simulink model "TempMeasure"  (R2014a)
settings: configuration reference "AR_Drone_ConfigSet" (kept outside this file)
libraries: simulink x6, AR_Drone_2_Library x2
settings Model: SimulationMode=external  ExtModeTrigDuration=480000  Creator=darenlee  LastModifiedBy=darenlee

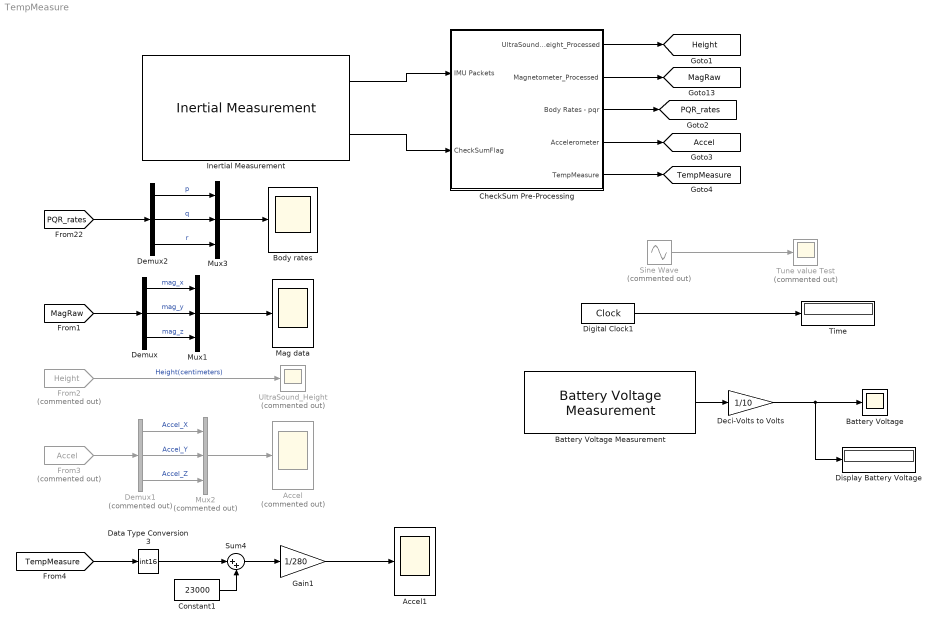
== system TempMeasure ==
  Accel : Scope  Commented=on
      settings: ShowLegends=on  TimeRange=100  YMin=2000  YMax=2550  SaveName=Accel
  Accel1 : Scope
      settings: ShowLegends=on  TimeRange=200  YMin=39  YMax=43.5  SaveName=TempMeasure
  Battery Voltage : Scope
      settings: YMin=12.3575  YMax=12.4  SaveName=Voltage_Measure
  Battery Voltage Measurement : AR_Drone_2_Library/Battery Voltage Measurement  SFunctionSpec=void BatteryMeasure_step(single y1[1])  SampleTime=0.01
  Body rates : Scope
      settings: ShowLegends=on  TimeRange=200  YMin=-45  YMax=45  SaveName=Gyro
  CheckSum Pre-Processing : Subsystem
  Constant1 : Constant  Value=23000  OutDataTypeStr=int16
  Data Type Conversion3 : DataTypeConversion  OutDataTypeStr=int16
  Deci-Volts to Volts : Gain  Gain=1/10
  Demux : Demux  Outputs=3
  Demux1 : Demux  Commented=on  Outputs=3
  Demux2 : Demux  Outputs=3
  Digital Clock1 : DigitalClock  SampleTime=0.1
  Display Battery Voltage : Display
  From2 : From  Commented=on  GotoTag=Height  TagVisibility=global
  From3 : From  Commented=on  GotoTag=Accel  TagVisibility=global
  Gain1 : Gain  Gain=1/280  OutDataTypeStr=double
  Inertial Measurement : AR_Drone_2_Library/Inertial Measurement  Ts=1/400
  Mag data : Scope
      settings: ShowLegends=on  TimeRange=100  YMin=-125  YMax=150  SaveName=MagData
  Mux1 : Mux  Inputs=3
  Mux2 : Mux  Commented=on  Inputs=3
  Mux3 : Mux  Inputs=3
  Sine Wave : Sin  Commented=on  SineType=Sample based  Amplitude=6  Bias=-1  Samples=1000  SampleTime=0.01
  Sum4 : Sum  Inputs=|++
  Time : Display
  Tune value Test : Scope  Commented=on
      settings: YMin=-35  SaveName=UltraSound_Measure2
  UltraSound_Height : Scope  Commented=on
      settings: YMin=0  YMax=18
  tag scope: Accel=global, Height=global, MagRaw=global, PQR_rates=global, TempMeasure=global
  wires:
  Sine Wave/1 -> Tune value Test/1
  Digital Clock1/1 -> Time/1
  Inertial Measurement/1 -> CheckSum Pre-Processing/1(IMU Packets)
  Inertial Measurement/2 -> CheckSum Pre-Processing/2(CheckSumFlag)
  [MagRaw] -> Demux/1
  Demux/1 -> Mux1/1  "mag_x"
  Demux/2 -> Mux1/2  "mag_y"
  Demux/3 -> Mux1/3  "mag_z"
  Mux1/1 -> Mag data/1
  CheckSum Pre-Processing/1(UltraSoundHeight_Processed) -> [Height]
  Demux2/1 -> Mux3/1  "p"
  Demux2/2 -> Mux3/2  "q"
  Mux3/1 -> Body rates/1
  Demux2/3 -> Mux3/3  "r"
  [PQR_rates] -> Demux2/1
  From2/1 -> UltraSound_Height/1  "Height(centimeters)"
  Demux1/1 -> Mux2/1  "Accel_X"
  Demux1/2 -> Mux2/2  "Accel_Y"
  Mux2/1 -> Accel/1
  Demux1/3 -> Mux2/3  "Accel_Z"
  From3/1 -> Demux1/1
  CheckSum Pre-Processing/4(Accelerometer) -> [Accel]
  CheckSum Pre-Processing/3(Body Rates - pqr) -> [PQR_rates]
  CheckSum Pre-Processing/2(Magnetometer_Processed) -> [MagRaw]
  Battery Voltage Measurement/1 -> Deci-Volts to Volts/1
  Deci-Volts to Volts/1 -> Display Battery Voltage/1, Battery Voltage/1
  CheckSum Pre-Processing/5(TempMeasure) -> [TempMeasure]
  Data Type Conversion3/1 -> Sum4/1
  Constant1/1 -> Sum4/2
  Sum4/1 -> Gain1/1
  Gain1/1 -> Accel1/1
  [TempMeasure] -> Data Type Conversion3/1

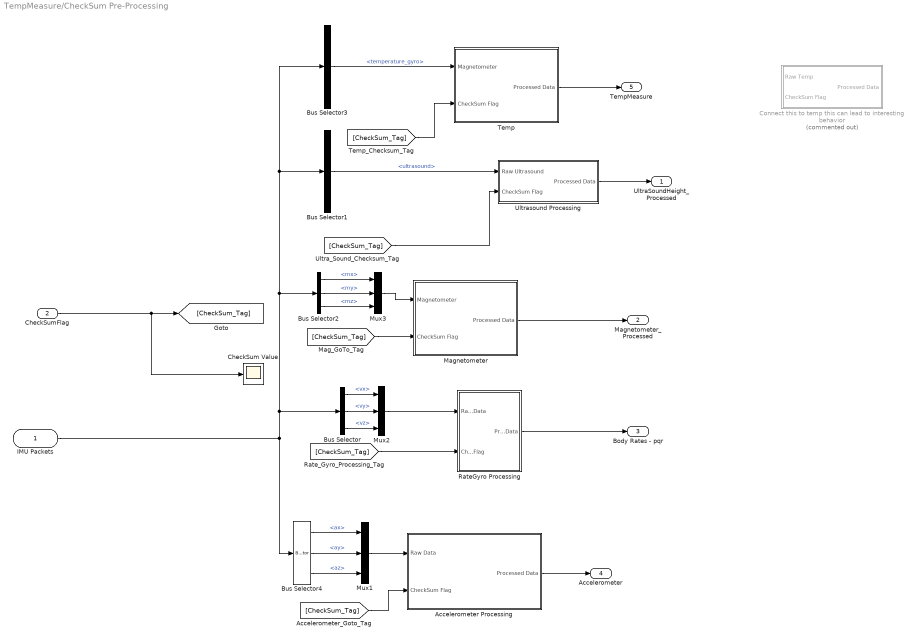
== system TempMeasure/CheckSum Pre-Processing ==
  IMU Packets : Inport
  CheckSumFlag : Inport  Port=2
  Accelerometer Processing : Subsystem
  Bus Selector : BusSelector  OutputSignals=vx,vy,vz
  Bus Selector1 : BusSelector  OutputSignals=ultrasound
  Bus Selector2 : BusSelector  OutputSignals=mx,my,mz
  Bus Selector3 : BusSelector  OutputSignals=temperature_gyro
  Bus Selector4 : BusSelector  OutputSignals=ax,ay,az
  CheckSum Value : Scope
      settings: YMin=0  YMax=2500  SaveName=CheckSum
  Connect this to temp this can lead to interesting behavior : Subsystem  Commented=on
  Magnetometer : Subsystem
  Mux1 : Mux  Inputs=3
  Mux2 : Mux  Inputs=3
  Mux3 : Mux  Inputs=3
  RateGyro Processing : Subsystem
  Temp : Subsystem
  Ultrasound Processing : Subsystem
  UltraSoundHeight_Processed : Outport
  Magnetometer_Processed : Outport  Port=2
  Body Rates - pqr : Outport  Port=3
  Accelerometer : Outport  Port=4
  TempMeasure : Outport  Port=5
  wires:
  Bus Selector1/1 -> Ultrasound Processing/1(Raw Ultrasound)  "<ultrasound>"
  CheckSumFlag/1 -> [CheckSum_Tag], CheckSum Value/1
  IMU Packets/1 -> Bus Selector/1, Bus Selector3/1, Bus Selector1/1, Bus Selector2/1, Bus Selector4/1
  Bus Selector4/1 -> Mux1/1  "<ax>"
  Bus Selector4/2 -> Mux1/2  "<ay>"
  Bus Selector4/3 -> Mux1/3  "<az>"
  Mux1/1 -> Accelerometer Processing/1(Raw Data)
  [CheckSum_Tag] -> Ultrasound Processing/2(CheckSum Flag)
  Accelerometer Processing/1(Processed Data) -> Accelerometer/1
  Bus Selector/1 -> Mux2/1  "<vx>"
  Bus Selector/2 -> Mux2/2  "<vy>"
  Bus Selector/3 -> Mux2/3  "<vz>"
  Mux2/1 -> RateGyro Processing/1(Raw Data)
  [CheckSum_Tag] -> RateGyro Processing/2(CheckSum Flag)
  RateGyro Processing/1(Processed Data) -> Body Rates - pqr/1
  Bus Selector2/1 -> Mux3/1  "<mx>"
  Bus Selector2/2 -> Mux3/2  "<my>"
  Bus Selector2/3 -> Mux3/3  "<mz>"
  Mux3/1 -> Magnetometer/1(Magnetometer)
  [CheckSum_Tag] -> Magnetometer/2(CheckSum Flag)
  Magnetometer/1(Processed Data) -> Magnetometer_Processed/1
  [CheckSum_Tag] -> Accelerometer Processing/2(CheckSum Flag)
  Ultrasound Processing/1(Processed Data) -> UltraSoundHeight_Processed/1
  Bus Selector3/1 -> Temp/1(Magnetometer)  "<temperature_gyro>"
  ? -> Connect this to temp this can lead to interesting behavior/2(CheckSum Flag)
  [CheckSum_Tag] -> Temp/2(CheckSum Flag)
  Temp/1(Processed Data) -> TempMeasure/1

== system TempMeasure/CheckSum Pre-Processing/Accelerometer Processing ==
  Raw Data : Inport
  CheckSum Flag : Inport  Port=2
  Calculate Accel Data : Subsystem  Commented=through
  CheckSum Correction : Subsystem
  Processed Data : Outport
  wires:
  CheckSum Flag/1 -> CheckSum Correction/2(CheckSumFlag)
  Raw Data/1 -> Calculate Accel Data/1(Raw Accel Data)
  CheckSum Correction/1(Pre-Processed Height) -> Processed Data/1
  Calculate Accel Data/1(Processed Accel Data) -> CheckSum Correction/1(CalculatedData)

== system TempMeasure/CheckSum Pre-Processing/Connect this to temp this can lead to interesting behavior ==
  note: '192.168.1.1' 1 17725
  Raw Temp : Inport
  CheckSum Flag : Inport  Port=2
  CheckSum Correction : Subsystem
  Display : Display
  Saturation1 : Saturate  UpperLimit=100e3  LowerLimit=0
  Processed Data : Outport
  wires:
  Raw Temp/1 -> CheckSum Correction/1(CalculatedData)
  CheckSum Flag/1 -> CheckSum Correction/2(CheckSumFlag)
  CheckSum Correction/1(Pre-Processed Height) -> Display/1, Saturation1/1
  Saturation1/1 -> Processed Data/1

== system TempMeasure/CheckSum Pre-Processing/Magnetometer ==
  Magnetometer : Inport
  CheckSum Flag : Inport  Port=2
  CheckSum Correction : Subsystem
  Display : Display
  Process Raw Mag Data : Subsystem  Commented=through
  Processed Data : Outport
  wires:
  CheckSum Flag/1 -> CheckSum Correction/2(CheckSumFlag)
  CheckSum Correction/1(Pre-Processed Data) -> Display/1, Processed Data/1
  Magnetometer/1 -> Process Raw Mag Data/1(Magnetometer)
  Process Raw Mag Data/1(ProcessedData) -> CheckSum Correction/1(CalculatedData)

== system TempMeasure/CheckSum Pre-Processing/RateGyro Processing ==
  Raw Data : Inport
  CheckSum Flag : Inport  Port=2
  CheckSum Correction : Subsystem
  Process Data : Subsystem  Commented=through
  Processed Data : Outport
  wires:
  CheckSum Flag/1 -> CheckSum Correction/2(CheckSumFlag)
  CheckSum Correction/1(Pre-Processed Height) -> Processed Data/1
  Raw Data/1 -> Process Data/1(Raw Data)
  Process Data/1(Processed Data) -> CheckSum Correction/1(CalculatedData)

== system TempMeasure/CheckSum Pre-Processing/Temp ==
  Magnetometer : Inport
  CheckSum Flag : Inport  Port=2
  CheckSum Correction : Subsystem
  Display : Display
  Process Raw Mag Data : Subsystem  Commented=through
  Processed Data : Outport
  wires:
  CheckSum Flag/1 -> CheckSum Correction/2(CheckSumFlag)
  CheckSum Correction/1(Pre-Processed Data) -> Display/1, Processed Data/1
  Magnetometer/1 -> Process Raw Mag Data/1(Magnetometer)
  Process Raw Mag Data/1(ProcessedData) -> CheckSum Correction/1(CalculatedData)

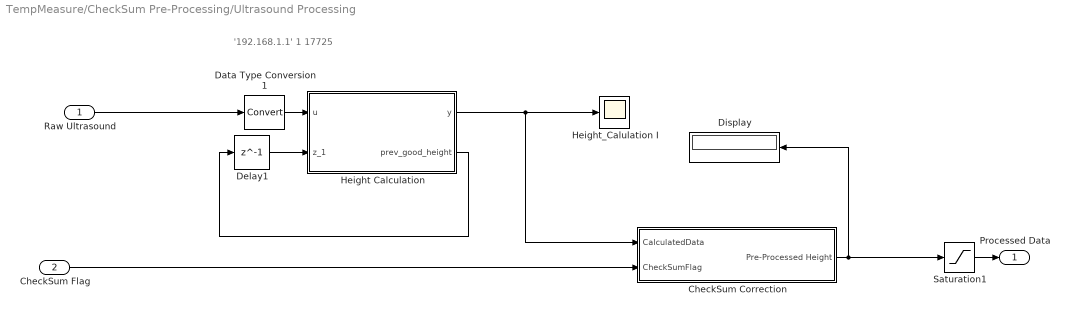
== system TempMeasure/CheckSum Pre-Processing/Ultrasound Processing ==
  note: '192.168.1.1' 1 17725
  Raw Ultrasound : Inport
  CheckSum Flag : Inport  Port=2
  CheckSum Correction : Subsystem
  Data Type Conversion1 : DataTypeConversion
  Delay1 : Delay  DelayLength=1  InitialCondition=0
  Display : Display
  Height Calculation : MATLAB Function  TreatAsAtomicUnit=on
  Height_Calulation I : Scope
      settings: TimeRange=622.5296442687759  YMin=0  YMax=300  SaveName=CalculatedHeight
  Saturation1 : Saturate  UpperLimit=100e3  LowerLimit=0
  Processed Data : Outport
  wires:
  Delay1/1 -> Height Calculation/2(z_1)
  Data Type Conversion1/1 -> Height Calculation/1(u)
  Height Calculation/2(prev_good_height) -> Delay1/1
  Raw Ultrasound/1 -> Data Type Conversion1/1
  Height Calculation/1(y) -> CheckSum Correction/1(CalculatedData), Height_Calulation I/1
  CheckSum Flag/1 -> CheckSum Correction/2(CheckSumFlag)
  CheckSum Correction/1(Pre-Processed Height) -> Display/1, Saturation1/1
  Saturation1/1 -> Processed Data/1

== system TempMeasure/CheckSum Pre-Processing/Accelerometer Processing/Calculate Accel Data ==
  Raw Accel Data : Inport
  Bias : Constant  Value=[0 4096 4096]
  Gain : Gain  Gain=[0.001953125, 0.001953125, 0.001953125]
  Neutral Bias : Constant  Value=[2048 2048 2048]
  Sum : Sum  Inputs=|-+
  Sum1 : Sum  Inputs=|+-
  Processed Accel Data : Outport
  wires:
  Raw Accel Data/1 -> Sum/1
  Sum1/1 -> Gain/1
  Gain/1 -> Processed Accel Data/1
  Sum/1 -> Sum1/1
  Neutral Bias/1 -> Sum1/2
  Bias/1 -> Sum/2

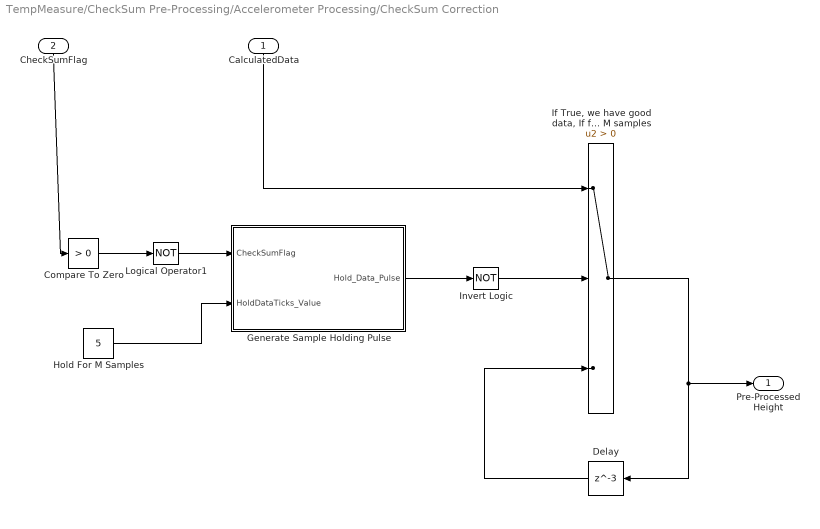
== system TempMeasure/CheckSum Pre-Processing/Accelerometer Processing/CheckSum Correction ==
  CalculatedData : Inport
  CheckSumFlag : Inport  Port=2
  Compare To Zero : simulink/Logic and Bit Operations/Compare To Zero  relop=>  OutDataTypeStr=boolean
  Delay : Delay  DelayLength=3  InitialCondition=0
  Generate Sample Holding Pulse : Subsystem
  Hold For M Samples : Constant  Value=5
  "If True, we have good data, If false, we have bad data, With bad data, use previous good data from N samples ago and hold it on that value for M samples" : Switch  Criteria=u2 > Threshold
  Invert Logic : Logic  Operator=NOT  AllPortsSameDT=off  OutDataTypeStr=boolean
  Logical Operator1 : Logic  Operator=NOT  AllPortsSameDT=off  OutDataTypeStr=boolean
  Pre-Processed Height : Outport
  wires:
  CheckSumFlag/1 -> Compare To Zero/1
  CalculatedData/1 -> "If True, we have good data, If false, we have bad data, With bad data, use previous good data from N samples ago and hold it on that value for M samples"/1
  "If True, we have good data, If false, we have bad data, With bad data, use previous good data from N samples ago and hold it on that value for M samples"/1 -> Pre-Processed Height/1, Delay/1
  Delay/1 -> "If True, we have good data, If false, we have bad data, With bad data, use previous good data from N samples ago and hold it on that value for M samples"/3
  Compare To Zero/1 -> Logical Operator1/1
  Generate Sample Holding Pulse/1(Hold_Data_Pulse) -> Invert Logic/1
  Logical Operator1/1 -> Generate Sample Holding Pulse/1(CheckSumFlag)
  Invert Logic/1 -> "If True, we have good data, If false, we have bad data, With bad data, use previous good data from N samples ago and hold it on that value for M samples"/2
  Hold For M Samples/1 -> Generate Sample Holding Pulse/2(HoldDataTicks_Value)

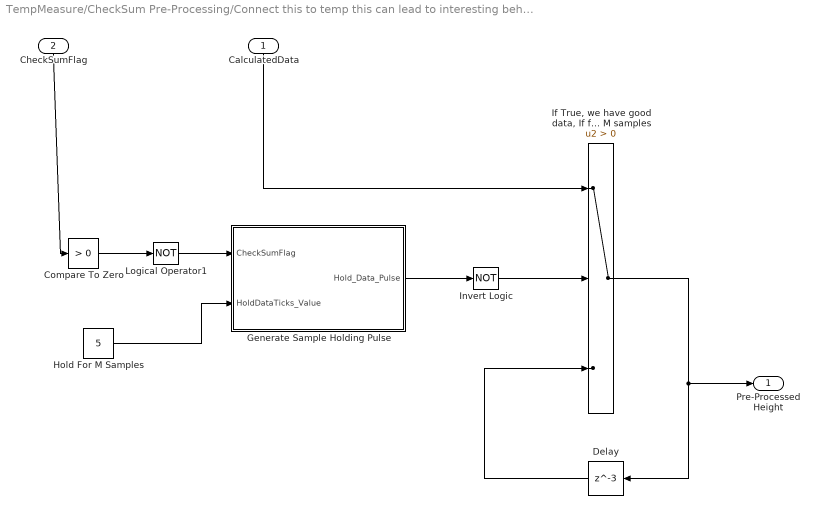
== system TempMeasure/CheckSum Pre-Processing/Connect this to temp this can lead to interesting behavior/CheckSum Correction ==
  CalculatedData : Inport
  CheckSumFlag : Inport  Port=2
  Compare To Zero : simulink/Logic and Bit Operations/Compare To Zero  relop=>  OutDataTypeStr=boolean
  Delay : Delay  DelayLength=3  InitialCondition=0
  Generate Sample Holding Pulse : Subsystem
  Hold For M Samples : Constant  Value=5
  "If True, we have good data, If false, we have bad data, With bad data, use previous good data from N samples ago and hold it on that value for M samples" : Switch  Criteria=u2 > Threshold
  Invert Logic : Logic  Operator=NOT  AllPortsSameDT=off  OutDataTypeStr=boolean
  Logical Operator1 : Logic  Operator=NOT  AllPortsSameDT=off  OutDataTypeStr=boolean
  Pre-Processed Height : Outport
  wires:
  CheckSumFlag/1 -> Compare To Zero/1
  CalculatedData/1 -> "If True, we have good data, If false, we have bad data, With bad data, use previous good data from N samples ago and hold it on that value for M samples"/1
  "If True, we have good data, If false, we have bad data, With bad data, use previous good data from N samples ago and hold it on that value for M samples"/1 -> Pre-Processed Height/1, Delay/1
  Delay/1 -> "If True, we have good data, If false, we have bad data, With bad data, use previous good data from N samples ago and hold it on that value for M samples"/3
  Compare To Zero/1 -> Logical Operator1/1
  Generate Sample Holding Pulse/1(Hold_Data_Pulse) -> Invert Logic/1
  Logical Operator1/1 -> Generate Sample Holding Pulse/1(CheckSumFlag)
  Invert Logic/1 -> "If True, we have good data, If false, we have bad data, With bad data, use previous good data from N samples ago and hold it on that value for M samples"/2
  Hold For M Samples/1 -> Generate Sample Holding Pulse/2(HoldDataTicks_Value)

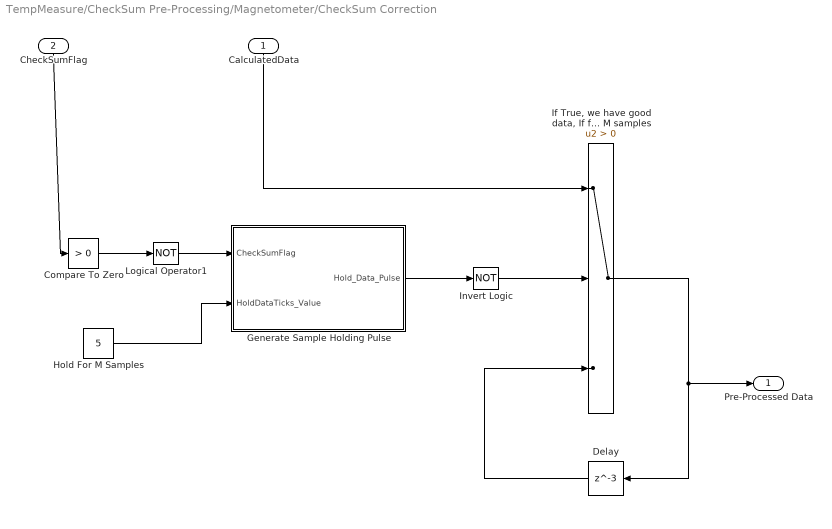
== system TempMeasure/CheckSum Pre-Processing/Magnetometer/CheckSum Correction ==
  CalculatedData : Inport
  CheckSumFlag : Inport  Port=2
  Compare To Zero : simulink/Logic and Bit Operations/Compare To Zero  relop=>  OutDataTypeStr=boolean
  Delay : Delay  DelayLength=3  InitialCondition=0
  Generate Sample Holding Pulse : Subsystem
  Hold For M Samples : Constant  Value=5
  "If True, we have good data, If false, we have bad data, With bad data, use previous good data from N samples ago and hold it on that value for M samples" : Switch  Criteria=u2 > Threshold
  Invert Logic : Logic  Operator=NOT  AllPortsSameDT=off  OutDataTypeStr=boolean
  Logical Operator1 : Logic  Operator=NOT  AllPortsSameDT=off  OutDataTypeStr=boolean
  Pre-Processed Data : Outport
  wires:
  CheckSumFlag/1 -> Compare To Zero/1
  CalculatedData/1 -> "If True, we have good data, If false, we have bad data, With bad data, use previous good data from N samples ago and hold it on that value for M samples"/1
  "If True, we have good data, If false, we have bad data, With bad data, use previous good data from N samples ago and hold it on that value for M samples"/1 -> Pre-Processed Data/1, Delay/1
  Delay/1 -> "If True, we have good data, If false, we have bad data, With bad data, use previous good data from N samples ago and hold it on that value for M samples"/3
  Compare To Zero/1 -> Logical Operator1/1
  Generate Sample Holding Pulse/1(Hold_Data_Pulse) -> Invert Logic/1
  Logical Operator1/1 -> Generate Sample Holding Pulse/1(CheckSumFlag)
  Invert Logic/1 -> "If True, we have good data, If false, we have bad data, With bad data, use previous good data from N samples ago and hold it on that value for M samples"/2
  Hold For M Samples/1 -> Generate Sample Holding Pulse/2(HoldDataTicks_Value)

== system TempMeasure/CheckSum Pre-Processing/Magnetometer/Process Raw Mag Data ==
  note: magnetometer[ 0 ] = - ( float ) navdata.mx ;
      | magnetometer[ 1 ] = ( float ) navdata.my ;
      | magnetometer[ 2 ] = - ( float ) navdata.mz ;
      | const float Sensitivity[ 3 ] = { 0.0071492608 , 0.0070882491 , 0.0074057781 } ;
      | const float Neutral[ 3 ] = { 118.0 , - 65.0 , 110.0 } ;
  Magnetometer : Inport
  Bias : Constant  Value=[ 118.0, -65.0, 110.0 ]
  Sum : Sum  Inputs=|+-
  postGain : Gain  Gain=[0.0071492608, 0.0070882491, 0.0074057781]
  preGain : Gain  Gain=[-1 1 -1]
  ProcessedData : Outport
  wires:
  postGain/1 -> ProcessedData/1
  Magnetometer/1 -> preGain/1
  Sum/1 -> postGain/1
  preGain/1 -> Sum/1
  Bias/1 -> Sum/2

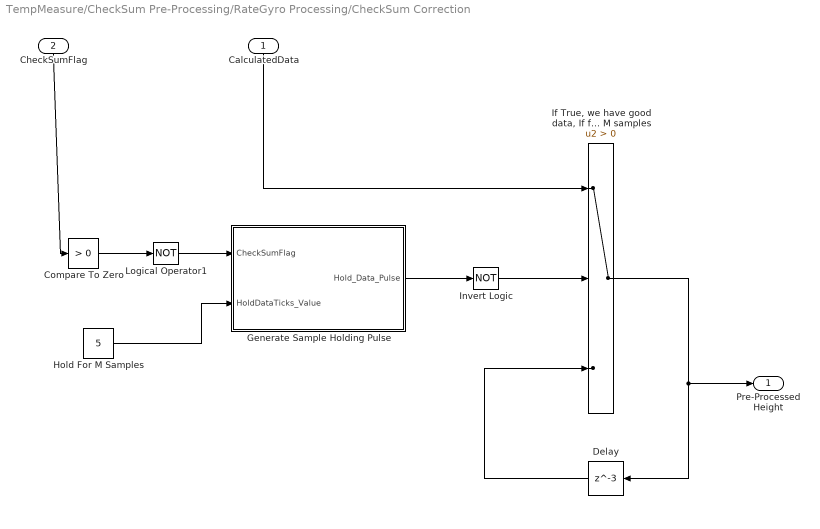
== system TempMeasure/CheckSum Pre-Processing/RateGyro Processing/CheckSum Correction ==
  CalculatedData : Inport
  CheckSumFlag : Inport  Port=2
  Compare To Zero : simulink/Logic and Bit Operations/Compare To Zero  relop=>  OutDataTypeStr=boolean
  Delay : Delay  DelayLength=3  InitialCondition=0
  Generate Sample Holding Pulse : Subsystem
  Hold For M Samples : Constant  Value=5  SampleTime=-1
  "If True, we have good data, If false, we have bad data, With bad data, use previous good data from N samples ago and hold it on that value for M samples" : Switch  Criteria=u2 > Threshold
  Invert Logic : Logic  Operator=NOT  AllPortsSameDT=off  OutDataTypeStr=boolean
  Logical Operator1 : Logic  Operator=NOT  AllPortsSameDT=off  OutDataTypeStr=boolean
  Pre-Processed Height : Outport
  wires:
  CheckSumFlag/1 -> Compare To Zero/1
  CalculatedData/1 -> "If True, we have good data, If false, we have bad data, With bad data, use previous good data from N samples ago and hold it on that value for M samples"/1
  "If True, we have good data, If false, we have bad data, With bad data, use previous good data from N samples ago and hold it on that value for M samples"/1 -> Pre-Processed Height/1, Delay/1
  Delay/1 -> "If True, we have good data, If false, we have bad data, With bad data, use previous good data from N samples ago and hold it on that value for M samples"/3
  Compare To Zero/1 -> Logical Operator1/1
  Generate Sample Holding Pulse/1(Hold_Data_Pulse) -> Invert Logic/1
  Logical Operator1/1 -> Generate Sample Holding Pulse/1(CheckSumFlag)
  Invert Logic/1 -> "If True, we have good data, If false, we have bad data, With bad data, use previous good data from N samples ago and hold it on that value for M samples"/2
  Hold For M Samples/1 -> Generate Sample Holding Pulse/2(HoldDataTicks_Value)

== system TempMeasure/CheckSum Pre-Processing/RateGyro Processing/Process Data ==
  note: const float Sensitivity[ 3 ] = { 0.0609 , 0.0609 , 0.0609 } ;
      | const float Neutral[ 3 ] = { 0.0 , 0.0 , 0.0 } ;
      | const int16_t Offset[ 3 ] = { - 73 , 14 , - 13 } ;
      | const int16_t Noises[ 3 ] = { 35 , 35 , 15 } ;
      |
      | int16_t vRaws[ 3 ] = {
      | Navdata :: IMU :: Gyroscope :: getRawX (),
      | Navdata :: IMU :: Gyroscope :: getRawY (),
      | Navdata :: IMU :: Gyroscope :: getRawZ ()
      | } ;
      |
      | gyroscope[i] = vRaws[i] * Gyroscope :: Sensitivity[i] * M_PI / 180.0 ;
  Raw Data : Inport
  Constant : Constant  Value=[0.0, 0.0, 0.0]
  Gain : Gain  Gain=[0.0609, 0.0609, 0.0609]
  Sum : Sum  Inputs=|++
  Processed Data : Outport
  wires:
  Sum/1 -> Gain/1
  Gain/1 -> Processed Data/1
  Constant/1 -> Sum/2
  Raw Data/1 -> Sum/1

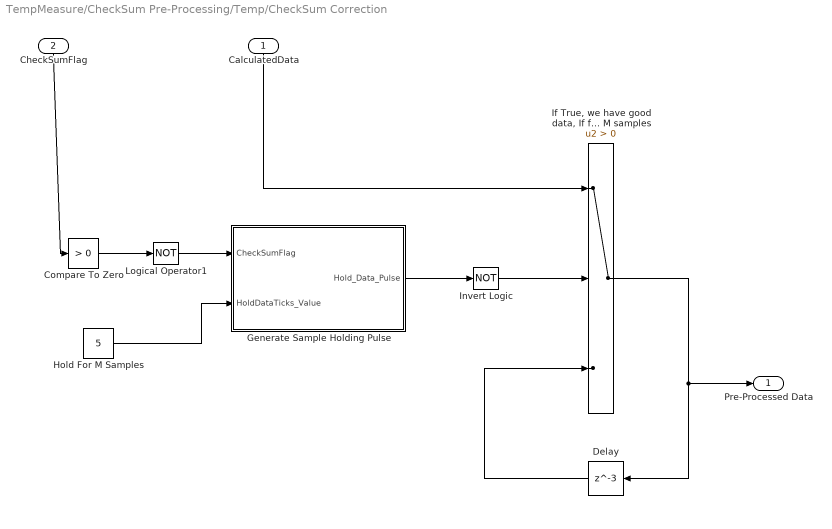
== system TempMeasure/CheckSum Pre-Processing/Temp/CheckSum Correction ==
  CalculatedData : Inport
  CheckSumFlag : Inport  Port=2
  Compare To Zero : simulink/Logic and Bit Operations/Compare To Zero  relop=>  OutDataTypeStr=boolean
  Delay : Delay  DelayLength=3  InitialCondition=0
  Generate Sample Holding Pulse : Subsystem
  Hold For M Samples : Constant  Value=5
  "If True, we have good data, If false, we have bad data, With bad data, use previous good data from N samples ago and hold it on that value for M samples" : Switch  Criteria=u2 > Threshold
  Invert Logic : Logic  Operator=NOT  AllPortsSameDT=off  OutDataTypeStr=boolean
  Logical Operator1 : Logic  Operator=NOT  AllPortsSameDT=off  OutDataTypeStr=boolean
  Pre-Processed Data : Outport
  wires:
  CheckSumFlag/1 -> Compare To Zero/1
  CalculatedData/1 -> "If True, we have good data, If false, we have bad data, With bad data, use previous good data from N samples ago and hold it on that value for M samples"/1
  "If True, we have good data, If false, we have bad data, With bad data, use previous good data from N samples ago and hold it on that value for M samples"/1 -> Pre-Processed Data/1, Delay/1
  Delay/1 -> "If True, we have good data, If false, we have bad data, With bad data, use previous good data from N samples ago and hold it on that value for M samples"/3
  Compare To Zero/1 -> Logical Operator1/1
  Generate Sample Holding Pulse/1(Hold_Data_Pulse) -> Invert Logic/1
  Logical Operator1/1 -> Generate Sample Holding Pulse/1(CheckSumFlag)
  Invert Logic/1 -> "If True, we have good data, If false, we have bad data, With bad data, use previous good data from N samples ago and hold it on that value for M samples"/2
  Hold For M Samples/1 -> Generate Sample Holding Pulse/2(HoldDataTicks_Value)

== system TempMeasure/CheckSum Pre-Processing/Temp/Process Raw Mag Data ==
  note: magnetometer[ 0 ] = - ( float ) navdata.mx ;
      | magnetometer[ 1 ] = ( float ) navdata.my ;
      | magnetometer[ 2 ] = - ( float ) navdata.mz ;
      | const float Sensitivity[ 3 ] = { 0.0071492608 , 0.0070882491 , 0.0074057781 } ;
      | const float Neutral[ 3 ] = { 118.0 , - 65.0 , 110.0 } ;
  Magnetometer : Inport
  Bias : Constant  Value=[ 118.0, -65.0, 110.0 ]
  Sum : Sum  Inputs=|+-
  postGain : Gain  Gain=[0.0071492608, 0.0070882491, 0.0074057781]
  preGain : Gain  Gain=[-1 1 -1]
  ProcessedData : Outport
  wires:
  postGain/1 -> ProcessedData/1
  Magnetometer/1 -> preGain/1
  Sum/1 -> postGain/1
  preGain/1 -> Sum/1
  Bias/1 -> Sum/2

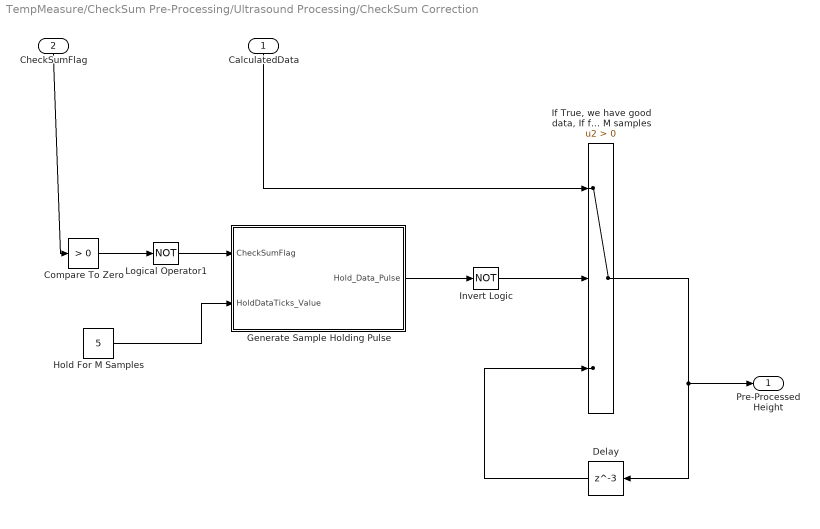
== system TempMeasure/CheckSum Pre-Processing/Ultrasound Processing/CheckSum Correction ==
  CalculatedData : Inport
  CheckSumFlag : Inport  Port=2
  Compare To Zero : simulink/Logic and Bit Operations/Compare To Zero  relop=>  OutDataTypeStr=boolean
  Delay : Delay  DelayLength=3  InitialCondition=0
  Generate Sample Holding Pulse : Subsystem
  Hold For M Samples : Constant  Value=5
  "If True, we have good data, If false, we have bad data, With bad data, use previous good data from N samples ago and hold it on that value for M samples" : Switch  Criteria=u2 > Threshold
  Invert Logic : Logic  Operator=NOT  AllPortsSameDT=off  OutDataTypeStr=boolean
  Logical Operator1 : Logic  Operator=NOT  AllPortsSameDT=off  OutDataTypeStr=boolean
  Pre-Processed Height : Outport
  wires:
  CheckSumFlag/1 -> Compare To Zero/1
  CalculatedData/1 -> "If True, we have good data, If false, we have bad data, With bad data, use previous good data from N samples ago and hold it on that value for M samples"/1
  "If True, we have good data, If false, we have bad data, With bad data, use previous good data from N samples ago and hold it on that value for M samples"/1 -> Pre-Processed Height/1, Delay/1
  Delay/1 -> "If True, we have good data, If false, we have bad data, With bad data, use previous good data from N samples ago and hold it on that value for M samples"/3
  Compare To Zero/1 -> Logical Operator1/1
  Generate Sample Holding Pulse/1(Hold_Data_Pulse) -> Invert Logic/1
  Logical Operator1/1 -> Generate Sample Holding Pulse/1(CheckSumFlag)
  Invert Logic/1 -> "If True, we have good data, If false, we have bad data, With bad data, use previous good data from N samples ago and hold it on that value for M samples"/2
  Hold For M Samples/1 -> Generate Sample Holding Pulse/2(HoldDataTicks_Value)

== system TempMeasure/CheckSum Pre-Processing/Accelerometer Processing/CheckSum Correction/Generate Sample Holding Pulse ==
  CheckSumFlag : Inport
  HoldDataTicks_Value : Inport  Port=2
  Chart : Stateflow chart  TreatAsAtomicUnit=on
  Constant2 : Constant
  Logical Operator1 : Logic  AllPortsSameDT=off  OutDataTypeStr=boolean
  Transition Logic Detection : Subsystem
  Hold_Data_Pulse : Outport
  wires:
  Constant2/1 -> Logical Operator1/1
  Logical Operator1/1 -> Hold_Data_Pulse/1
  Chart/1(output) -> Logical Operator1/2
  Transition Logic Detection/1(Transition Detect) -> Chart/1(if_transition)
  CheckSumFlag/1 -> Transition Logic Detection/1(Input)
  HoldDataTicks_Value/1 -> Chart/2(HoldDataTicks)

== system TempMeasure/CheckSum Pre-Processing/Connect this to temp this can lead to interesting behavior/CheckSum Correction/Generate Sample Holding Pulse ==
  CheckSumFlag : Inport
  HoldDataTicks_Value : Inport  Port=2
  Chart : Stateflow chart  TreatAsAtomicUnit=on
  Constant2 : Constant
  Logical Operator1 : Logic  AllPortsSameDT=off  OutDataTypeStr=boolean
  Transition Logic Detection : Subsystem
  Hold_Data_Pulse : Outport
  wires:
  Constant2/1 -> Logical Operator1/1
  Logical Operator1/1 -> Hold_Data_Pulse/1
  Chart/1(output) -> Logical Operator1/2
  Transition Logic Detection/1(Transition Detect) -> Chart/1(if_transition)
  CheckSumFlag/1 -> Transition Logic Detection/1(Input)
  HoldDataTicks_Value/1 -> Chart/2(HoldDataTicks)

== system TempMeasure/CheckSum Pre-Processing/Magnetometer/CheckSum Correction/Generate Sample Holding Pulse ==
  CheckSumFlag : Inport
  HoldDataTicks_Value : Inport  Port=2
  Chart : Stateflow chart  TreatAsAtomicUnit=on
  Constant2 : Constant
  Logical Operator1 : Logic  AllPortsSameDT=off  OutDataTypeStr=boolean
  Transition Logic Detection : Subsystem
  Hold_Data_Pulse : Outport
  wires:
  Constant2/1 -> Logical Operator1/1
  Logical Operator1/1 -> Hold_Data_Pulse/1
  Chart/1(output) -> Logical Operator1/2
  Transition Logic Detection/1(Transition Detect) -> Chart/1(if_transition)
  CheckSumFlag/1 -> Transition Logic Detection/1(Input)
  HoldDataTicks_Value/1 -> Chart/2(HoldDataTicks)

== system TempMeasure/CheckSum Pre-Processing/RateGyro Processing/CheckSum Correction/Generate Sample Holding Pulse ==
  CheckSumFlag : Inport
  HoldDataTicks_Value : Inport  Port=2
  Chart : Stateflow chart  TreatAsAtomicUnit=on
  Constant2 : Constant
  Logical Operator1 : Logic  AllPortsSameDT=off  OutDataTypeStr=boolean
  Transition Logic Detection : Subsystem
  Hold_Data_Pulse : Outport
  wires:
  Constant2/1 -> Logical Operator1/1
  Logical Operator1/1 -> Hold_Data_Pulse/1
  Chart/1(output) -> Logical Operator1/2
  Transition Logic Detection/1(Transition Detect) -> Chart/1(if_transition)
  CheckSumFlag/1 -> Transition Logic Detection/1(Input)
  HoldDataTicks_Value/1 -> Chart/2(HoldDataTicks)

== system TempMeasure/CheckSum Pre-Processing/Temp/CheckSum Correction/Generate Sample Holding Pulse ==
  CheckSumFlag : Inport
  HoldDataTicks_Value : Inport  Port=2
  Chart : Stateflow chart  TreatAsAtomicUnit=on
  Constant2 : Constant
  Logical Operator1 : Logic  AllPortsSameDT=off  OutDataTypeStr=boolean
  Transition Logic Detection : Subsystem
  Hold_Data_Pulse : Outport
  wires:
  Constant2/1 -> Logical Operator1/1
  Logical Operator1/1 -> Hold_Data_Pulse/1
  Chart/1(output) -> Logical Operator1/2
  Transition Logic Detection/1(Transition Detect) -> Chart/1(if_transition)
  CheckSumFlag/1 -> Transition Logic Detection/1(Input)
  HoldDataTicks_Value/1 -> Chart/2(HoldDataTicks)

== system TempMeasure/CheckSum Pre-Processing/Ultrasound Processing/CheckSum Correction/Generate Sample Holding Pulse ==
  CheckSumFlag : Inport
  HoldDataTicks_Value : Inport  Port=2
  Chart : Stateflow chart  TreatAsAtomicUnit=on
  Constant2 : Constant
  Logical Operator1 : Logic  AllPortsSameDT=off  OutDataTypeStr=boolean
  Transition Logic Detection : Subsystem
  Hold_Data_Pulse : Outport
  wires:
  Constant2/1 -> Logical Operator1/1
  Logical Operator1/1 -> Hold_Data_Pulse/1
  Chart/1(output) -> Logical Operator1/2
  Transition Logic Detection/1(Transition Detect) -> Chart/1(if_transition)
  CheckSumFlag/1 -> Transition Logic Detection/1(Input)
  HoldDataTicks_Value/1 -> Chart/2(HoldDataTicks)

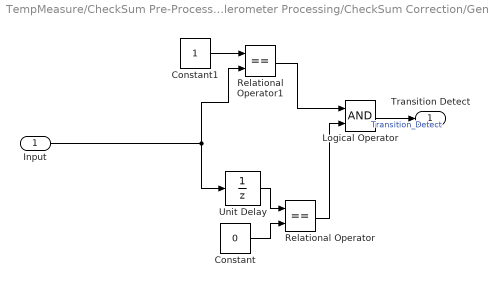
== system TempMeasure/CheckSum Pre-Processing/Accelerometer Processing/CheckSum Correction/Generate Sample Holding Pulse/Transition Logic Detection ==
  Input : Inport
  Constant : Constant  Value=0
  Constant1 : Constant
  Logical Operator : Logic  AllPortsSameDT=off  OutDataTypeStr=boolean
  Relational Operator : RelationalOperator  Operator===  OutDataTypeStr=boolean
  Relational Operator1 : RelationalOperator  Operator===  OutDataTypeStr=boolean
  Unit Delay : UnitDelay  SampleTime=-1
  Transition Detect : Outport
  wires:
  Relational Operator1/1 -> Logical Operator/1
  Unit Delay/1 -> Relational Operator/1
  Input/1 -> Relational Operator1/2, Unit Delay/1
  Relational Operator/1 -> Logical Operator/2
  Constant/1 -> Relational Operator/2
  Constant1/1 -> Relational Operator1/1
  Logical Operator/1 -> Transition Detect/1  "Transition_Detect"

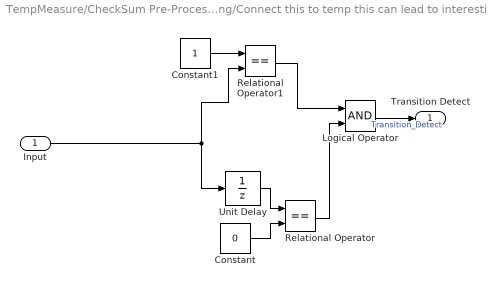
== system TempMeasure/CheckSum Pre-Processing/Connect this to temp this can lead to interesting behavior/CheckSum Correction/Generate Sample Holding Pulse/Transition Logic Detection ==
  Input : Inport
  Constant : Constant  Value=0
  Constant1 : Constant
  Logical Operator : Logic  AllPortsSameDT=off  OutDataTypeStr=boolean
  Relational Operator : RelationalOperator  Operator===  OutDataTypeStr=boolean
  Relational Operator1 : RelationalOperator  Operator===  OutDataTypeStr=boolean
  Unit Delay : UnitDelay  SampleTime=-1
  Transition Detect : Outport
  wires:
  Relational Operator1/1 -> Logical Operator/1
  Unit Delay/1 -> Relational Operator/1
  Input/1 -> Relational Operator1/2, Unit Delay/1
  Relational Operator/1 -> Logical Operator/2
  Constant/1 -> Relational Operator/2
  Constant1/1 -> Relational Operator1/1
  Logical Operator/1 -> Transition Detect/1  "Transition_Detect"

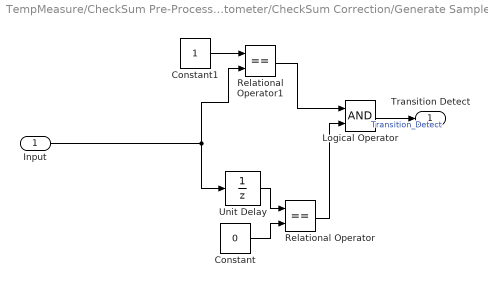
== system TempMeasure/CheckSum Pre-Processing/Magnetometer/CheckSum Correction/Generate Sample Holding Pulse/Transition Logic Detection ==
  Input : Inport
  Constant : Constant  Value=0
  Constant1 : Constant
  Logical Operator : Logic  AllPortsSameDT=off  OutDataTypeStr=boolean
  Relational Operator : RelationalOperator  Operator===  OutDataTypeStr=boolean
  Relational Operator1 : RelationalOperator  Operator===  OutDataTypeStr=boolean
  Unit Delay : UnitDelay  SampleTime=-1
  Transition Detect : Outport
  wires:
  Relational Operator1/1 -> Logical Operator/1
  Unit Delay/1 -> Relational Operator/1
  Input/1 -> Relational Operator1/2, Unit Delay/1
  Relational Operator/1 -> Logical Operator/2
  Constant/1 -> Relational Operator/2
  Constant1/1 -> Relational Operator1/1
  Logical Operator/1 -> Transition Detect/1  "Transition_Detect"

== system TempMeasure/CheckSum Pre-Processing/RateGyro Processing/CheckSum Correction/Generate Sample Holding Pulse/Transition Logic Detection ==
  Input : Inport
  Constant : Constant  Value=0
  Constant1 : Constant
  Logical Operator : Logic  AllPortsSameDT=off  OutDataTypeStr=boolean
  Relational Operator : RelationalOperator  Operator===  OutDataTypeStr=boolean
  Relational Operator1 : RelationalOperator  Operator===  OutDataTypeStr=boolean
  Unit Delay : UnitDelay  SampleTime=-1
  Transition Detect : Outport
  wires:
  Relational Operator1/1 -> Logical Operator/1
  Unit Delay/1 -> Relational Operator/1
  Input/1 -> Relational Operator1/2, Unit Delay/1
  Relational Operator/1 -> Logical Operator/2
  Constant/1 -> Relational Operator/2
  Constant1/1 -> Relational Operator1/1
  Logical Operator/1 -> Transition Detect/1  "Transition_Detect"

== system TempMeasure/CheckSum Pre-Processing/Temp/CheckSum Correction/Generate Sample Holding Pulse/Transition Logic Detection ==
  Input : Inport
  Constant : Constant  Value=0
  Constant1 : Constant
  Logical Operator : Logic  AllPortsSameDT=off  OutDataTypeStr=boolean
  Relational Operator : RelationalOperator  Operator===  OutDataTypeStr=boolean
  Relational Operator1 : RelationalOperator  Operator===  OutDataTypeStr=boolean
  Unit Delay : UnitDelay  SampleTime=-1
  Transition Detect : Outport
  wires:
  Relational Operator1/1 -> Logical Operator/1
  Unit Delay/1 -> Relational Operator/1
  Input/1 -> Relational Operator1/2, Unit Delay/1
  Relational Operator/1 -> Logical Operator/2
  Constant/1 -> Relational Operator/2
  Constant1/1 -> Relational Operator1/1
  Logical Operator/1 -> Transition Detect/1  "Transition_Detect"

== system TempMeasure/CheckSum Pre-Processing/Ultrasound Processing/CheckSum Correction/Generate Sample Holding Pulse/Transition Logic Detection ==
  Input : Inport
  Constant : Constant  Value=0
  Constant1 : Constant
  Logical Operator : Logic  AllPortsSameDT=off  OutDataTypeStr=boolean
  Relational Operator : RelationalOperator  Operator===  OutDataTypeStr=boolean
  Relational Operator1 : RelationalOperator  Operator===  OutDataTypeStr=boolean
  Unit Delay : UnitDelay  SampleTime=-1
  Transition Detect : Outport
  wires:
  Relational Operator1/1 -> Logical Operator/1
  Unit Delay/1 -> Relational Operator/1
  Input/1 -> Relational Operator1/2, Unit Delay/1
  Relational Operator/1 -> Logical Operator/2
  Constant/1 -> Relational Operator/2
  Constant1/1 -> Relational Operator1/1
  Logical Operator/1 -> Transition Detect/1  "Transition_Detect"

== matlab function TempMeasure/CheckSum Pre-Processing/Ultrasound Processing/Height Calculation ==
  data: u input double; y output double; prev_good_height output double; z_1 input double
function [y,prev_good_height] = fcn(u,z_1)
%#codegen



if u<10000
    
    height = ((u - 880) /26.553);
    prev_good_height = height;
else
    
%     height = u;
%     prev_good_height = height;
    height =  z_1;
    prev_good_height = z_1; 
end

y = height;

== stateflow chart TempMeasure/CheckSum Pre-Processing/Accelerometer Processing/CheckSum Correction/Generate Sample Holding Pulse/Chart ==
  state Begin_State0
    entry: output =0;
  state Begin_State
    entry: output =1;
  state End_State
    entry: output=0;
  (default) -> Begin_State0
  Begin_State0 -> Begin_State : [if_transition==1]
  Begin_State -> End_State [order 1] : after(HoldDataTicks,tick)
  End_State -> Begin_State : [if_transition==1]
  Begin_State -> Begin_State [order 2] : [if_transition==1]
  data: output output; if_transition input; HoldDataTicks input

== stateflow chart TempMeasure/CheckSum Pre-Processing/RateGyro Processing/CheckSum Correction/Generate Sample Holding Pulse/Chart ==
  state Begin_State0
    entry: output =0;
  state Begin_State
    entry: output =1;
  state End_State
    entry: output=0;
  (default) -> Begin_State0
  Begin_State0 -> Begin_State : [if_transition==1]
  Begin_State -> End_State [order 1] : after(HoldDataTicks,tick)
  End_State -> Begin_State : [if_transition==1]
  Begin_State -> Begin_State [order 2] : [if_transition==1]
  data: output output; if_transition input; HoldDataTicks input

== stateflow chart TempMeasure/CheckSum Pre-Processing/Ultrasound Processing/CheckSum Correction/Generate Sample Holding Pulse/Chart ==
  state Begin_State0
    entry: output =0;
  state Begin_State
    entry: output =1;
  state End_State
    entry: output=0;
  (default) -> Begin_State0
  Begin_State0 -> Begin_State : [if_transition==1]
  Begin_State -> End_State [order 1] : after(HoldDataTicks,tick)
  End_State -> Begin_State : [if_transition==1]
  Begin_State -> Begin_State [order 2] : [if_transition==1]
  data: output output; if_transition input; HoldDataTicks input

== stateflow chart TempMeasure/CheckSum Pre-Processing/Magnetometer/CheckSum Correction/Generate Sample Holding Pulse/Chart ==
  state Begin_State0
    entry: output =0;
  state Begin_State
    entry: output =1;
  state End_State
    entry: output=0;
  (default) -> Begin_State0
  Begin_State0 -> Begin_State : [if_transition==1]
  Begin_State -> End_State [order 1] : after(HoldDataTicks,tick)
  End_State -> Begin_State : [if_transition==1]
  Begin_State -> Begin_State [order 2] : [if_transition==1]
  data: output output; if_transition input; HoldDataTicks input

== stateflow chart TempMeasure/CheckSum Pre-Processing/Connect this to temp this can lead to interesting behavior/CheckSum Correction/Generate Sample Holding Pulse/Chart ==
  state Begin_State0
    entry: output =0;
  state Begin_State
    entry: output =1;
  state End_State
    entry: output=0;
  (default) -> Begin_State0
  Begin_State0 -> Begin_State : [if_transition==1]
  Begin_State -> End_State [order 1] : after(HoldDataTicks,tick)
  End_State -> Begin_State : [if_transition==1]
  Begin_State -> Begin_State [order 2] : [if_transition==1]
  data: output output; if_transition input; HoldDataTicks input

== stateflow chart TempMeasure/CheckSum Pre-Processing/Temp/CheckSum Correction/Generate Sample Holding Pulse/Chart ==
  state Begin_State0
    entry: output =0;
  state Begin_State
    entry: output =1;
  state End_State
    entry: output=0;
  (default) -> Begin_State0
  Begin_State0 -> Begin_State : [if_transition==1]
  Begin_State -> End_State [order 1] : after(HoldDataTicks,tick)
  End_State -> Begin_State : [if_transition==1]
  Begin_State -> Begin_State [order 2] : [if_transition==1]
  data: output output; if_transition input; HoldDataTicks input
